simulink model "v_cruise_control"  (R2022b)
settings: Solver=VariableStepAuto  StartTime=0.0  StopTime=10.0  RelTol=1e-3
settings Model: Creator=Tamer  LastModifiedBy=Tamer
settings SolverCC: ZeroCrossControl=DisableAll  AlgebraicLoopSolver=TrustRegion
settings DataIOCC: SaveOutput=off  SaveTime=off
settings DebuggingCC: UnconnectedInputMsg=warning  UnconnectedOutputMsg=warning  UnconnectedLineMsg=warning  SFMachineParentedDataDiag=warning
settings ModelReferenceCC: EnableRefExpFcnMdlSchedulingChecks=on
settings GRTTargetCC: CombineOutputUpdateFcns=off  MatFileLogging=off

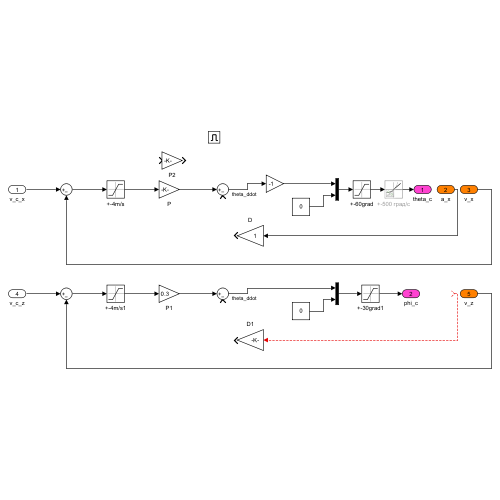
[thumbnail: Simulink's stored preview of the top-level diagram]
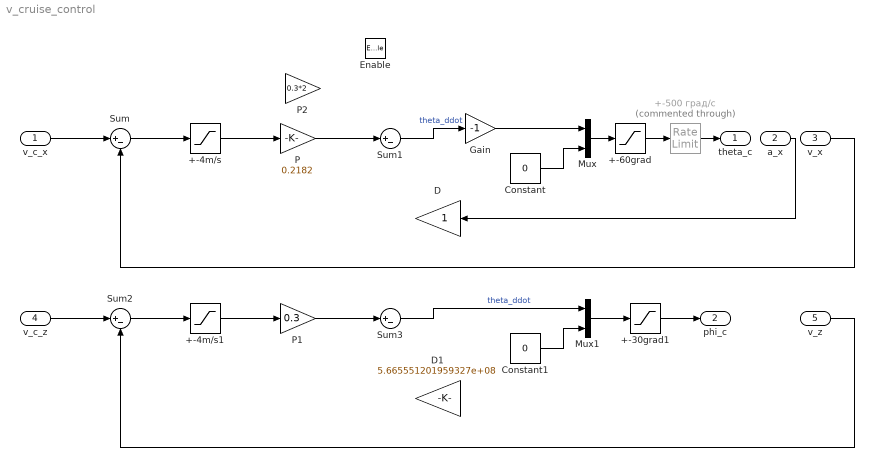
== system v_cruise_control ==
  v_c_x : Inport
  a_x : Inport  Port=2
  v_x : Inport  Port=3
  v_c_z : Inport  Port=4
  v_z : Inport  Port=5
  Enable : EnablePort
  +-30grad1 : Saturate  UpperLimit=deg2rad(40)  LowerLimit=-deg2rad(40)
  +-4m/s : Saturate  UpperLimit=4  LowerLimit=-4
  +-4m/s1 : Saturate  UpperLimit=4  LowerLimit=-4
  +-500 град/с : RateLimiter  Commented=through  RisingSlewLimit=deg2rad(500)  FallingSlewLimit=-deg2rad(500)  SampleTimeMode=inherited
  +-60grad : Saturate  UpperLimit=deg2rad(60)  LowerLimit=-deg2rad(60)
  Constant : Constant  Value=0
  Constant1 : Constant  Value=0
  D : Gain
  D1 : Gain  Gain=5.665551201959327e+08
  Gain : Gain  Gain=-1
  Mux : Mux  Inputs=2
  Mux1 : Mux  Inputs=2
  P : Gain  Gain=0.2182
  P1 : Gain  Gain=0.3
  P2 : Gain  Gain=0.3*2
  Sum{,1..3} (4 alike) : Sum  Inputs=|+-
  theta_c : Outport
  phi_c : Outport  Port=2
  wires:
  P/1 -> Sum1/1
  a_x/1 -> D/1
  v_c_x/1 -> Sum/1
  Sum/1 -> +-4m/s/1
  v_x/1 -> Sum/2
  +-4m/s/1 -> P/1
  Constant/1 -> Mux/2
  Mux/1 -> +-60grad/1
  Sum1/1 -> Gain/1  "theta_ddot"
  Gain/1 -> Mux/1
  Mux1/1 -> +-30grad1/1
  Sum2/1 -> +-4m/s1/1
  Constant1/1 -> Mux1/2
  P1/1 -> Sum3/1
  v_c_z/1 -> Sum2/1
  Sum3/1 -> Mux1/1  "theta_ddot"
  +-30grad1/1 -> phi_c/1
  v_z/1 -> Sum2/2
  +-4m/s1/1 -> P1/1
  ? -> D1/1
  +-60grad/1 -> +-500 град/с/1
  +-500 град/с/1 -> theta_c/1
